simulink model "Planteamientos"  (R2024b)
settings: Solver=VariableStepAuto  StartTime=0.0  StopTime=10.0  RelTol=1e-3
libraries: SignalEditorBlockLib x1

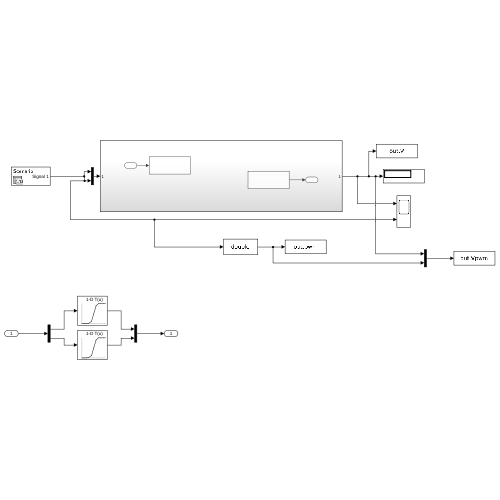
[thumbnail: Simulink's stored preview of the top-level diagram]
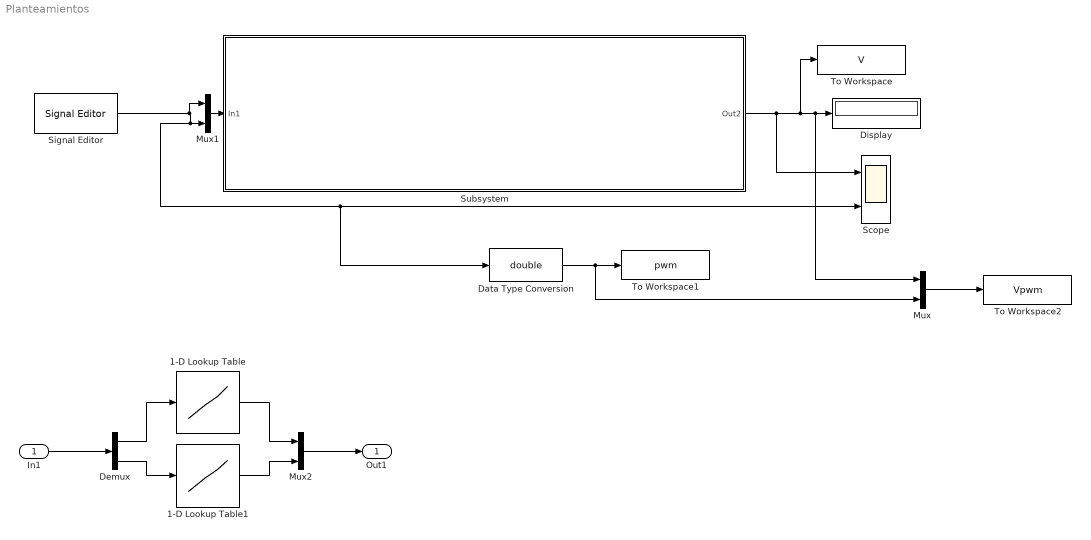
== system Planteamientos ==
  In1 : Inport
  1-D Lookup Table : Lookup_n-D  NumberOfTableDimensions=1  BreakpointsForDimension1=[-5:5]  Table=tanh([-5:5])  InternalRulePriority=Speed  RndMeth=Simplest
  1-D Lookup Table1 : Lookup_n-D  NumberOfTableDimensions=1  BreakpointsForDimension1=[-5:5]  Table=tanh([-5:5])  InternalRulePriority=Speed  RndMeth=Simplest
  Data Type Conversion : DataTypeConversion  OutDataTypeStr=double  SaturateOnIntegerOverflow=off  RndMeth=Floor
  Demux : Demux  Outputs=2
  Display : Display
  Mux : Mux  Inputs=2
  Mux1 : Mux  Inputs=2
  Mux2 : Mux  Inputs=2
  Scope : Scope  NumInputPorts=2
  Signal Editor : SignalEditorBlockLib/Signal Editor  FileName=untitled.mat  ActiveScenario=Scenario  ActiveSignal=Signal 1  IsBus=off  OutputBusObjectStr=Bus: BusObject  SampleTime=0  Interpolate=off  ZeroCross=off  OutputAfterFinalValue=Setting to zero  Unit=inherit  PreserveSignalName=on  ApplySigPropsToAllScenarios=on  ApplySigPropsToAllSignals=off
  Subsystem : Subsystem
  To Workspace : ToWorkspace  VariableName=V  SampleTime=-1
      settings: Save2DSignal=2-D array (concatenate along first dimension)
  To Workspace1 : ToWorkspace  VariableName=pwm  SampleTime=-1
      settings: Save2DSignal=2-D array (concatenate along first dimension)
  To Workspace2 : ToWorkspace  VariableName=Vpwm  SampleTime=-1
      settings: Save2DSignal=2-D array (concatenate along first dimension)
  Out1 : Outport
  wires:
  Subsystem/1(Out2) -> Scope/1, To Workspace/1, Mux/1, Display/1
  Signal Editor/1 -> Mux1/1, Mux1/2, Data Type Conversion/1, Scope/2
  Data Type Conversion/1 -> Mux/2, To Workspace1/1
  Mux/1 -> To Workspace2/1
  Mux1/1 -> Subsystem/1(In1)
  In1/1 -> Demux/1
  Demux/1 -> 1-D Lookup Table/1
  1-D Lookup Table/1 -> Mux2/1
  Mux2/1 -> Out1/1
  Demux/2 -> 1-D Lookup Table1/1
  1-D Lookup Table1/1 -> Mux2/2

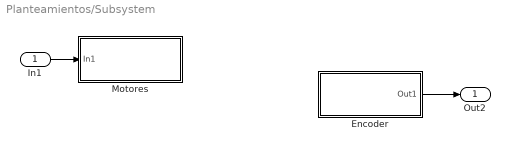
== system Planteamientos/Subsystem ==
  In1 : Inport
  Encoder : Subsystem
  Motores : Subsystem
  Out2 : Outport
  wires:
  In1/1 -> Motores/1(In1)
  Encoder/1(Out1) -> Out2/1

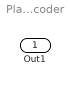
== system Planteamientos/Subsystem/Encoder ==
  Out1 : Outport

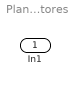
== system Planteamientos/Subsystem/Motores ==
  In1 : Inport
